simulink model "Sim_ControladorLQRdiscreto"  (R2024a)
settings: Solver=ode15s  StartTime=0.0  StopTime=10  MaxStep=.0001  RelTol=1e-3
values from neighbouring files (symbols this model uses):
  deg_inicial = 5    [DisenControl.m]
  h = 0.001    [DisenControl.m]
  K = lqr(mA, mB, Q, R)    [DisenControl.m]
  Kd = dlqr(mG,mH,Q,R)    [DisenControl.m]
  mA = [       0,   1,        0,                 0 ... (first row only)    [Parametros_Proyecto.m]
  mB = [0 ... (first row only)    [Parametros_Proyecto.m]
  mC = eye(4)    [Parametros_Proyecto.m]
  mD = [0; 0; 0; 0]    [Parametros_Proyecto.m]
settings Model: Creator=isposzax  LastModifiedBy=alen2
settings ConfigComp: CovBoundaryAbsTol=1.0e-5

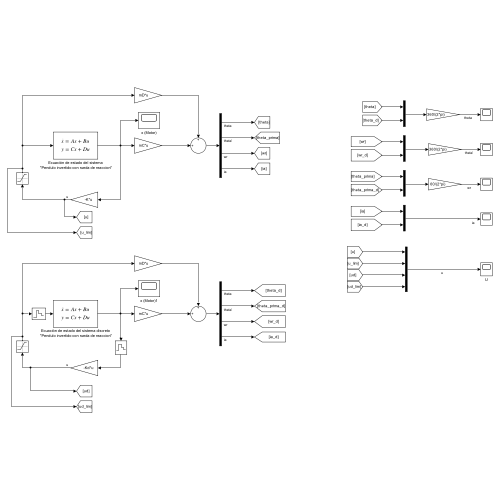
[thumbnail: Simulink's stored preview of the top-level diagram]
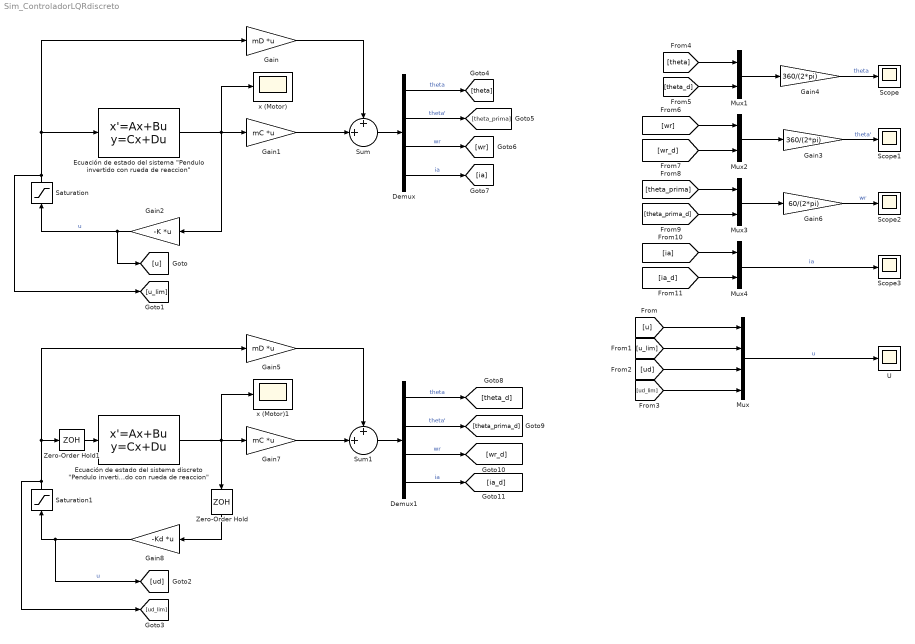
== system Sim_ControladorLQRdiscreto ==
  Demux : Demux
  Demux1 : Demux
  "Ecuación de estado del sistema \"Pendulo invertido con rueda de reaccion\"" : StateSpace  A=mA  B=mB  C=mC  D=mD  InitialCondition=[deg_inicial*pi/180 0 0 0]
  "Ecuación de estado del sistema discreto \"Pendulo invertido con rueda de reaccion\"" : StateSpace  A=mA  B=mB  C=mC  D=mD  InitialCondition=[deg_inicial*pi/180 0 0 0]
  Gain : Gain  Gain=mD  Multiplication=Matrix(K*u)
  Gain1 : Gain  Gain=mC  Multiplication=Matrix(K*u)
  Gain2 : Gain  Gain=-K  Multiplication=Matrix(K*u)
  Gain3 : Gain  Gain=360/(2*pi)
  Gain4 : Gain  Gain=360/(2*pi)
  Gain5 : Gain  Gain=mD  Multiplication=Matrix(K*u)
  Gain6 : Gain  Gain=60/(2*pi)
  Gain7 : Gain  Gain=mC  Multiplication=Matrix(K*u)
  Gain8 : Gain  Gain=-Kd  Multiplication=Matrix(K*u)
  Mux : Mux
  Mux{1..4} (4 alike) : Mux  Inputs=2
  Saturation : Saturate  UpperLimit=12  LowerLimit=-12
  Saturation1 : Saturate  UpperLimit=12  LowerLimit=-12
  Scope{,1..3} (4 alike) : Scope
  Sum : Sum  Inputs=++|
  Sum1 : Sum  Inputs=++|
  U : Scope
  Zero-Order Hold : ZeroOrderHold  SampleTime=h
  Zero-Order Hold1 : ZeroOrderHold  SampleTime=h
  x (Motor) : Scope
  x (Motor)1 : Scope
  wires:
  Gain2/1 -> [u], Saturation/1  "u"
  "Ecuación de estado del sistema \"Pendulo invertido con rueda de reaccion\""/1 -> x (Motor)/1, Gain2/1, Gain1/1
  Gain1/1 -> Sum/2
  Gain/1 -> Sum/1
  Sum/1 -> Demux/1
  Gain4/1 -> Scope/1  "theta"
  Gain3/1 -> Scope1/1  "theta'"
  Gain6/1 -> Scope2/1  "wr"
  Saturation/1 -> "Ecuación de estado del sistema \"Pendulo invertido con rueda de reaccion\""/1, Gain/1, [u_lim]
  Sum1/1 -> Demux1/1
  Gain5/1 -> Sum1/1
  Gain7/1 -> Sum1/2
  Gain8/1 -> [ud], Saturation1/1  "u"
  Demux/1 -> [theta]  "theta"
  Demux/2 -> [theta_prima]  "theta'"
  Demux/3 -> [wr]  "wr"
  Demux/4 -> [ia]  "ia"
  Demux1/1 -> [theta_d]  "theta"
  Demux1/2 -> [theta_prima_d]  "theta'"
  Demux1/3 -> [wr_d]  "wr"
  Demux1/4 -> [ia_d]  "ia"
  Mux/1 -> U/1  "u"
  [u] -> Mux/1
  [u_lim] -> Mux/2
  [ud] -> Mux/3
  [ud_lim] -> Mux/4
  [theta_d] -> Mux1/2
  [theta] -> Mux1/1
  Mux1/1 -> Gain4/1
  [wr] -> Mux2/1
  [wr_d] -> Mux2/2
  Mux2/1 -> Gain3/1
  [theta_prima_d] -> Mux3/2
  [theta_prima] -> Mux3/1
  Mux3/1 -> Gain6/1
  [ia] -> Mux4/1
  [ia_d] -> Mux4/2
  Mux4/1 -> Scope3/1  "ia"
  "Ecuación de estado del sistema discreto \"Pendulo invertido con rueda de reaccion\""/1 -> Zero-Order Hold/1, Gain7/1, x (Motor)1/1
  Saturation1/1 -> Zero-Order Hold1/1, Gain5/1, [ud_lim]
  Zero-Order Hold/1 -> Gain8/1
  Zero-Order Hold1/1 -> "Ecuación de estado del sistema discreto \"Pendulo invertido con rueda de reaccion\""/1
